simulink model "mylib_R2016b"  (R2016b)
settings: Solver=FixedStepAuto  StartTime=0.0  StopTime=10.0  RelTol=1e-3  SampleTimeConstraint=STIndependent
undefined symbols (not defined in the file or in its folder): In2, Mask_inport, Mask_outport, Out2
libraries: simulink x9
(part 1 of 2)
settings Model: Creator=Colin  LastModifiedBy=zhoutinglin
settings SimscapeCC: SimscapeNormalizeSystem=off

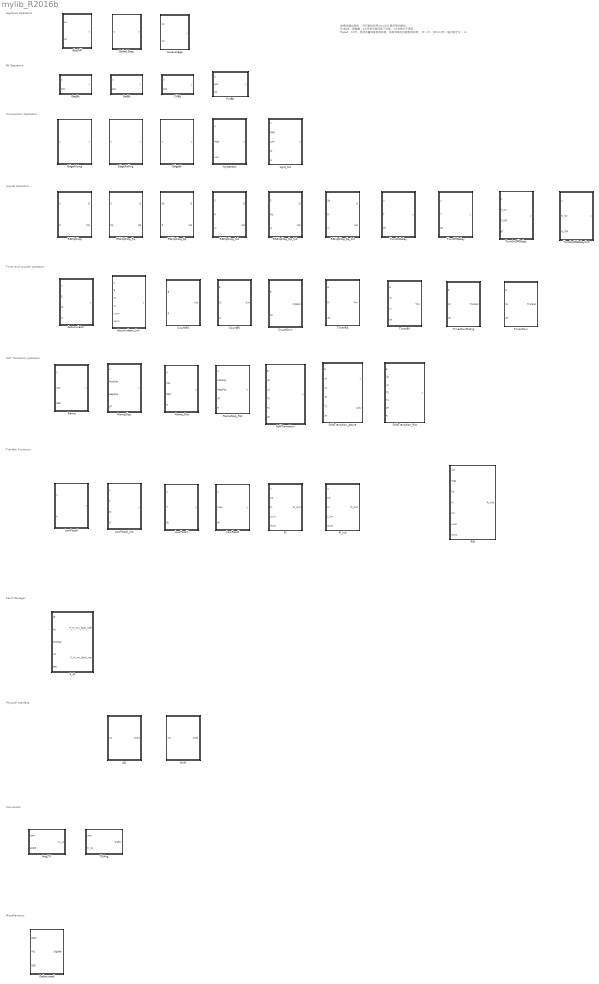
== system mylib_R2016b ==
  note: 库模块建立原则：
      | 尽可能的利用simulink里自带的模块；
      | Enable，逻辑量，=1时表示激活某个功能；=0时表示不激活，
      | Reset，=1时，将状态量恢复到初始值，或者将输出恢复到初始值；
      | IC，IV：当IC=1时，输出等于IV；
      |
      | 3.
  note: Algebraic Operators
  note: Bit Operators
  note: Comparision Operators
  note: Logical Operators
  note: Timer and counter operators
  note: Soft Transitioin operators
  note: Transfer Functions
  note: Fault Manager
  note: Physical Interface
  note: Conversion
  note: Miscellaneous
  AD : Subsystem
  AbsDiff : Subsystem
  Accumulator : Subsystem
  Accumulator_Lim : Subsystem
  Ang2Ti : Subsystem
  ClrBit : Subsystem
  CountDwn : Subsystem
  CountEV : Subsystem
  CountRE : Subsystem
  Debounced : Subsystem
  Delta1Step : Subsystem
  EdgeBi : Subsystem
  EdgeFalling : Subsystem
  EdgeRising : Subsystem
  F_M : Subsystem
  GetBit : Subsystem
  Hyst_Init : Subsystem
  Hysteresis : Subsystem
  LowPassF : Subsystem
  LowPassK : Subsystem
  LowPassK_Init : Subsystem
  LowPassT : Subsystem
  NVM : Subsystem
  PI : Subsystem
  PID : Subsystem
  PI_Init : Subsystem
  PutBit : Subsystem
  RSFilpFlop : Subsystem
  RSFilpFlop_Init : Subsystem
  RSFilpFlop_Rp : Subsystem
  RSFilpFlop_Rp_Init : Subsystem
  RSFilpFlop_Sp : Subsystem
  RSFilpFlop_Sp_Init : Subsystem
  Ramp : Subsystem
  RampSlop : Subsystem
  RampSlop_Rst : Subsystem
  Ramp_Rst : Subsystem
  SetBit : Subsystem
  SoftTransition : Subsystem
  SoftTransition_Active : Subsystem
  SoftTransition_Rst : Subsystem
  Ti2Ang : Subsystem
  TimerDwn : Subsystem
  TimerDwnRetrig : Subsystem
  TimerEV : Subsystem
  TimerRE : Subsystem
  TurnOffDelay : Subsystem
  TurnOnDelay : Subsystem
  TurnOnOffDelay : Subsystem
  TurnOnOffDelayCnt : Subsystem
  twoAverage : Subsystem

== system mylib_R2016b/AD ==
  In1 : Inport
  Out1 : Outport

== system mylib_R2016b/AbsDiff ==
  u1 : Inport
  u2 : Inport  Port=2
  Abs : Abs  RndMeth=Round  SaturateOnIntegerOverflow=on
  Subtract : Sum  Inputs=+-  RndMeth=Round  SaturateOnIntegerOverflow=on  InputSameDT=on  OutDataTypeStr=Inherit: Same as first input
  y : Outport
  wires:
  Abs/1 -> y/1
  u1/1 -> Subtract/1
  u2/1 -> Subtract/2
  Subtract/1 -> Abs/1

== system mylib_R2016b/Accumulator ==
  u : Inport
  E : Inport  Port=2  OutDataTypeStr=boolean
  IC : Inport  Port=3  OutDataTypeStr=boolean
  IV : Inport  Port=4
  Add : Sum  RndMeth=Round  SaturateOnIntegerOverflow=on  InputSameDT=on  OutDataTypeStr=Inherit: Same as first input
  Delay : Delay  DelayLength=1  InitialConditionSource=Input port  ExternalReset=Rising
      settings: InputPortMap=u0,r5,p4
  Switch : Switch  Criteria=u2 ~= 0  InputSameDT=on
  Switch1 : Switch  Criteria=u2 ~= 0  InputSameDT=on
  y : Outport
  wires:
  E/1 -> Delay/2, Switch/2
  Switch1/1 -> Delay/1, y/1
  IC/1 -> Switch1/2
  IV/1 -> Switch1/1
  Switch/1 -> Switch1/3
  u/1 -> Delay/3, Add/1
  Delay/1 -> Switch/3, Add/2
  Add/1 -> Switch/1

== system mylib_R2016b/Accumulator_Lim ==
  u : Inport
  E : Inport  Port=2  OutDataTypeStr=boolean
  IC : Inport  Port=3  OutDataTypeStr=boolean
  IV : Inport  Port=4
  LLim : Inport  Port=5
  HLim : Inport  Port=6
  Add : Sum  RndMeth=Round  SaturateOnIntegerOverflow=on  InputSameDT=on  OutDataTypeStr=Inherit: Same as first input
  Delay : Delay  DelayLength=1  InitialConditionSource=Input port  ExternalReset=Rising
      settings: InputPortMap=u0,r5,p4
  Relational Operator : RelationalOperator  Operator=<=  OutDataTypeStr=boolean  RndMeth=Simplest  InputSameDT=on
  Relational Operator1 : RelationalOperator  OutDataTypeStr=boolean  RndMeth=Simplest  InputSameDT=on
  Switch : Switch  Criteria=u2 ~= 0  InputSameDT=on
  Switch1 : Switch  Criteria=u2 ~= 0  InputSameDT=on
  Switch2 : Switch  Criteria=u2 ~= 0
  Switch3 : Switch  Criteria=u2 ~= 0
  y : Outport
  wires:
  E/1 -> Delay/2, Switch/2
  IC/1 -> Switch1/2
  IV/1 -> Switch1/1
  u/1 -> Delay/3, Add/1
  Delay/1 -> Switch/3, Add/2
  Add/1 -> Switch/1
  Relational Operator1/1 -> Switch2/2
  LLim/1 -> Switch3/1, Relational Operator/2
  Relational Operator/1 -> Switch3/2
  HLim/1 -> Relational Operator1/2, Switch2/1
  Switch2/1 -> Switch3/3
  Switch/1 -> Switch1/3
  Switch1/1 -> Switch2/3, Relational Operator1/1, Relational Operator/1
  Switch3/1 -> Delay/1, y/1

== system mylib_R2016b/Ang2Ti ==
  rpm : Inport
  angle : Inport  Port=2
  Constant : Constant  Value=1000000  OutDataTypeStr=uint32
  Constant1 : Constant  Value=6  OutDataTypeStr=uint8
  Divide : Product  Inputs=*/  OutDataTypeStr=fixdt(1,32,10)  SaturateOnIntegerOverflow=on
  Divide1 : Product  Inputs=*/  OutDataTypeStr=fixdt(1,32,10)  SaturateOnIntegerOverflow=on
  Product : Product  OutDataTypeStr=Inherit: Inherit via back propagation  SaturateOnIntegerOverflow=on
  ti_us : Outport
  wires:
  rpm/1 -> Divide/2
  Constant/1 -> Divide/1
  Divide/1 -> Divide1/1
  Constant1/1 -> Divide1/2
  Divide1/1 -> Product/1
  angle/1 -> Product/2
  Product/1 -> ti_us/1

== system mylib_R2016b/ClrBit ==
  u : Inport
  pos : Inport  Port=2  OutDataTypeStr=uint8
  Bitwise Operator : simulink/Logic and Bit Operations/Bitwise Operator  logicop=AND  UseBitMask=off  NumInputPorts=2  BitMask=bin2dec('11011001')  BitMaskRealWorld=Stored Integer
  Bitwise Operator1 : simulink/Logic and Bit Operations/Bitwise Operator  logicop=NOT  UseBitMask=off  BitMask=bin2dec('11011001')  BitMaskRealWorld=Stored Integer
  Constant2 : Constant  OutDataTypeStr=Inherit: Inherit via back propagation
  Data Type Duplicate : DataTypeDuplicate  NumInputPorts=3
  Shift Arithmetic : ArithShift  BitShiftNumberSource=Input port  BitShiftNumber=8  BitShiftDirection=Left
      settings: InputPortMap=u0,p1
  y : Outport
  wires:
  pos/1 -> Shift Arithmetic/2
  Shift Arithmetic/1 -> Bitwise Operator1/1
  Constant2/1 -> Data Type Duplicate/2, Shift Arithmetic/1
  u/1 -> Data Type Duplicate/1, Bitwise Operator/1
  Bitwise Operator/1 -> Data Type Duplicate/3, y/1
  Bitwise Operator1/1 -> Bitwise Operator/2

== system mylib_R2016b/CountDwn ==
  E : Inport  OutDataTypeStr=boolean
  SV : Inport  Port=2
  Add : Sum  Inputs=+-  RndMeth=Round  SaturateOnIntegerOverflow=on  InputSameDT=on  OutDataTypeStr=Inherit: Same as first input
  Constant : Constant  OutDataTypeStr=Inherit: Inherit via back propagation
  Constant2 : Constant  Value=0  OutDataTypeStr=Inherit: Inherit via back propagation
  Delay : Delay  DelayLength=1  InitialConditionSource=Input port  ExternalReset=Rising
      settings: InputPortMap=u0,r5,p4
  Relational Operator : RelationalOperator  Operator=<=  OutDataTypeStr=boolean  RndMeth=Simplest  InputSameDT=on
  Switch : Switch  Criteria=u2 ~= 0  InputSameDT=on
  CntEnd : Outport  OutDataTypeStr=boolean
  wires:
  Add/1 -> Switch/1
  Switch/1 -> Delay/1, Relational Operator/1
  Delay/1 -> Switch/3, Add/1
  Constant/1 -> Add/2
  SV/1 -> Delay/3
  E/1 -> Switch/2, Delay/2
  Relational Operator/1 -> CntEnd/1
  Constant2/1 -> Relational Operator/2

== system mylib_R2016b/CountEV ==
  E : Inport  OutDataTypeStr=boolean
  IC : Inport  Port=2  OutDataTypeStr=boolean
  IV : Inport  Port=3
  Add : Sum  OutDataTypeStr=Inherit: Inherit via back propagation  RndMeth=Round  SaturateOnIntegerOverflow=on  InputSameDT=on
  Constant : Constant  OutDataTypeStr=Inherit: Inherit via back propagation
  Data Type Duplicate : DataTypeDuplicate
  Switch : Switch  Criteria=u2 ~= 0  OutDataTypeStr=Inherit: Inherit via back propagation  InputSameDT=on
  Switch1 : Switch  Criteria=u2 ~= 0  OutDataTypeStr=Inherit: Inherit via back propagation  InputSameDT=on
  Unit Delay : UnitDelay  SampleTime=-1
      settings: AttributesFormatString=InitialValue=%<InitialCondition>
  Cnt : Outport
  wires:
  E/1 -> Switch/2
  Add/1 -> Switch/1
  Switch1/1 -> Data Type Duplicate/2, Unit Delay/1, Cnt/1
  IC/1 -> Switch1/2
  IV/1 -> Data Type Duplicate/1, Switch1/1
  Switch/1 -> Switch1/3
  Constant/1 -> Add/1
  Unit Delay/1 -> Switch/3, Add/2

== system mylib_R2016b/CountRE ==
  E : Inport  OutDataTypeStr=boolean
  R : Inport  Port=2  OutDataTypeStr=boolean
  Add : Sum  OutDataTypeStr=Inherit: Inherit via back propagation  SaturateOnIntegerOverflow=on  InputSameDT=on
  Constant : Constant  OutDataTypeStr=Inherit: Inherit via back propagation
  Constant2 : Constant  Value=0  OutDataTypeStr=Inherit: Inherit via back propagation
  Switch : Switch  Criteria=u2 ~= 0  OutDataTypeStr=Inherit: Inherit via back propagation  InputSameDT=on
  Switch1 : Switch  Criteria=u2 ~= 0  OutDataTypeStr=Inherit: Inherit via back propagation  InputSameDT=on
  Unit Delay : UnitDelay  SampleTime=-1
      settings: AttributesFormatString=InitialValue=%<InitialCondition>
  Cnt : Outport
  wires:
  E/1 -> Switch/2
  Add/1 -> Switch/1
  Switch1/1 -> Unit Delay/1, Cnt/1
  R/1 -> Switch1/2
  Constant2/1 -> Switch1/1
  Switch/1 -> Switch1/3
  Constant/1 -> Add/1
  Unit Delay/1 -> Switch/3, Add/2

== system mylib_R2016b/Debounced ==
  SigIn : Inport  OutDataTypeStr=boolean
  INC : Inport  Port=2
  DEC : Inport  Port=3
  Add : Sum
  Constant : Constant  Value=65535
  Constant1 : Constant  Value=0  OutDataTypeStr=boolean
  Constant2 : Constant  OutDataTypeStr=boolean
  Relational Operator : RelationalOperator  OutDataTypeStr=boolean  RndMeth=Simplest
  Subtract : Sum  Inputs=+-
  Switch : Switch  Criteria=u2 ~= 0
  Switch1 : Switch  Criteria=u2 ~= 0
  Unit Delay : UnitDelay  SampleTime=-1
      settings: AttributesFormatString=InitialValue=%<InitialCondition>
  SigDeb : Outport  OutDataTypeStr=boolean
  wires:
  SigIn/1 -> Switch/2
  Switch/1 -> Unit Delay/1, Relational Operator/1
  Constant/1 -> Relational Operator/2
  Relational Operator/1 -> Switch1/2
  Switch1/1 -> SigDeb/1
  Constant1/1 -> Switch1/3
  Constant2/1 -> Switch1/1
  INC/1 -> Add/2
  Unit Delay/1 -> Subtract/1, Add/1
  Add/1 -> Switch/1
  Subtract/1 -> Switch/3
  DEC/1 -> Subtract/2

== system mylib_R2016b/Delta1Step ==
  u : Inport
  Delay : Delay  DelayLength=1  InitialConditionSource=Input port
      settings: InputPortMap=u0,p4
  Subtract : Sum  Inputs=+-  RndMeth=Round  SaturateOnIntegerOverflow=on  InputSameDT=on  OutDataTypeStr=Inherit: Same as first input
  y : Outport
  wires:
  u/1 -> Delay/1, Delay/2, Subtract/1
  Subtract/1 -> y/1
  Delay/1 -> Subtract/2

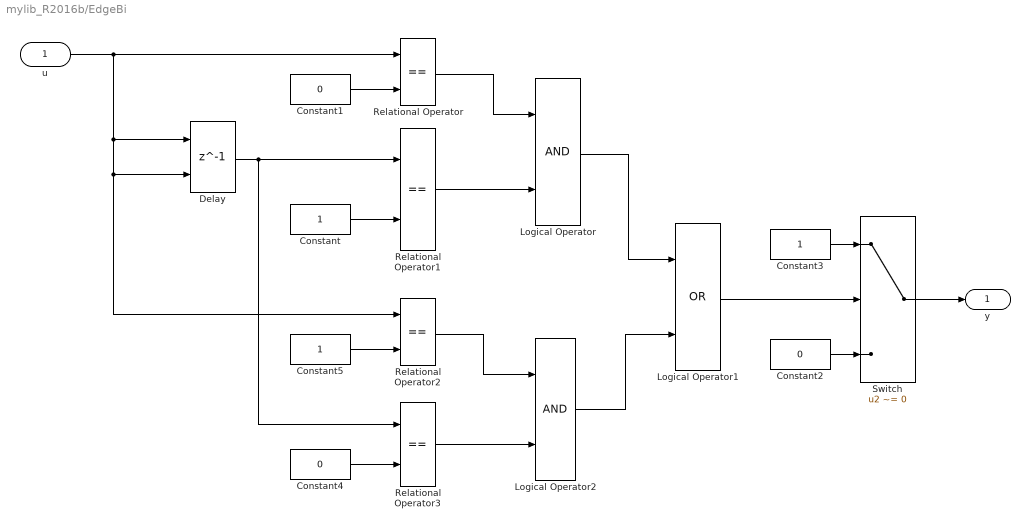
== system mylib_R2016b/EdgeBi ==
  u : Inport  OutDataTypeStr=boolean
  Constant : Constant  OutDataTypeStr=boolean
  Constant1 : Constant  Value=0  OutDataTypeStr=boolean
  Constant2 : Constant  Value=0  OutDataTypeStr=boolean
  Constant3 : Constant  OutDataTypeStr=boolean
  Constant4 : Constant  Value=0  OutDataTypeStr=boolean
  Constant5 : Constant  OutDataTypeStr=boolean
  Delay : Delay  DelayLength=1  InitialConditionSource=Input port
      settings: InputPortMap=u0,p4
  Logical Operator : Logic  AllPortsSameDT=off  OutDataTypeStr=boolean
  Logical Operator1 : Logic  Operator=OR  AllPortsSameDT=off  OutDataTypeStr=boolean
  Logical Operator2 : Logic  AllPortsSameDT=off  OutDataTypeStr=boolean
  Relational Operator{,1..3} (4 alike) : RelationalOperator  Operator===  OutDataTypeStr=boolean  RndMeth=Simplest
  Switch : Switch  Criteria=u2 ~= 0  InputSameDT=on
  y : Outport  OutDataTypeStr=boolean
  wires:
  Delay/1 -> Relational Operator3/1, Relational Operator1/1
  Switch/1 -> y/1
  Constant/1 -> Relational Operator1/2
  Constant1/1 -> Relational Operator/2
  Relational Operator1/1 -> Logical Operator/2
  Relational Operator/1 -> Logical Operator/1
  Constant2/1 -> Switch/3
  Constant3/1 -> Switch/1
  Logical Operator/1 -> Logical Operator1/1
  Logical Operator2/1 -> Logical Operator1/2
  u/1 -> Relational Operator2/1, Delay/2, Delay/1, Relational Operator/1
  Constant5/1 -> Relational Operator2/2
  Relational Operator2/1 -> Logical Operator2/1
  Constant4/1 -> Relational Operator3/2
  Relational Operator3/1 -> Logical Operator2/2
  Logical Operator1/1 -> Switch/2

== system mylib_R2016b/EdgeFalling ==
  u : Inport  OutDataTypeStr=boolean
  Constant : Constant  OutDataTypeStr=boolean
  Constant1 : Constant  Value=0  OutDataTypeStr=boolean
  Constant2 : Constant  Value=0  OutDataTypeStr=boolean
  Constant3 : Constant  OutDataTypeStr=boolean
  Delay : Delay  DelayLength=1  InitialConditionSource=Input port
      settings: InputPortMap=u0,p4
  Logical Operator : Logic  AllPortsSameDT=off  OutDataTypeStr=boolean
  Relational Operator : RelationalOperator  Operator===  OutDataTypeStr=boolean  RndMeth=Simplest
  Relational Operator1 : RelationalOperator  Operator===  OutDataTypeStr=boolean  RndMeth=Simplest
  Switch : Switch  Criteria=u2 ~= 0  InputSameDT=on
  y : Outport  OutDataTypeStr=boolean
  wires:
  Logical Operator/1 -> Switch/2
  Switch/1 -> y/1
  u/1 -> Delay/2, Delay/1, Relational Operator/1
  Constant1/1 -> Relational Operator/2
  Constant/1 -> Relational Operator1/2
  Delay/1 -> Relational Operator1/1
  Relational Operator/1 -> Logical Operator/1
  Relational Operator1/1 -> Logical Operator/2
  Constant2/1 -> Switch/3
  Constant3/1 -> Switch/1

== system mylib_R2016b/EdgeRising ==
  u : Inport  OutDataTypeStr=boolean
  Constant : Constant  Value=0  OutDataTypeStr=boolean
  Constant1 : Constant  OutDataTypeStr=boolean
  Constant2 : Constant  Value=0  OutDataTypeStr=boolean
  Constant3 : Constant  OutDataTypeStr=boolean
  Delay : Delay  DelayLength=1  InitialConditionSource=Input port
      settings: InputPortMap=u0,p4
  Logical Operator : Logic  AllPortsSameDT=off  OutDataTypeStr=boolean
  Relational Operator : RelationalOperator  Operator===  OutDataTypeStr=boolean  RndMeth=Simplest
  Relational Operator1 : RelationalOperator  Operator===  OutDataTypeStr=boolean  RndMeth=Simplest
  Switch : Switch  Criteria=u2 ~= 0  InputSameDT=on
  y : Outport  OutDataTypeStr=boolean
  wires:
  Logical Operator/1 -> Switch/2
  Switch/1 -> y/1
  u/1 -> Delay/1, Delay/2, Relational Operator/1
  Constant1/1 -> Relational Operator/2
  Constant/1 -> Relational Operator1/2
  Delay/1 -> Relational Operator1/1
  Relational Operator/1 -> Logical Operator/1
  Relational Operator1/1 -> Logical Operator/2
  Constant2/1 -> Switch/3
  Constant3/1 -> Switch/1

== system mylib_R2016b/F_M ==
  df : Inport  LibraryBlock=Mask_inport/In2  OutDataTypeStr=boolean
  frz : Inport  LibraryBlock=Mask_inport/In2  Port=2  OutDataTypeStr=boolean
  enClear : Inport  LibraryBlock=Mask_inport/In2  Port=3  OutDataTypeStr=boolean
  inc : Inport  LibraryBlock=Mask_inport/In2  Port=4  OutDataTypeStr=uint16
  dec : Inport  LibraryBlock=Mask_inport/In2  Port=5  OutDataTypeStr=uint16
  Soft : Subsystem
  rec : Subsystem
  F_M_xxx_fault_soft : Outport  LibraryBlock=Mask_outport/Out2  OutDataTypeStr=boolean  OutputWhenUnconnectedValue=0  VectorParamsAs1DForOutWhenUnconnected=off
  F_M_xxx_fault_rec : Outport  LibraryBlock=Mask_outport/Out2  Port=2  OutDataTypeStr=boolean  OutputWhenUnconnectedValue=0  VectorParamsAs1DForOutWhenUnconnected=off
  wires:
  inc/1 -> rec/4(inc)
  dec/1 -> rec/5(dec)
  Soft/1(F_M_xxx_fault_soft) -> F_M_xxx_fault_soft/1
  rec/1(F_M_xxx_fault_rec) -> F_M_xxx_fault_rec/1
  df/1 -> rec/1(df), Soft/1(df)
  frz/1 -> rec/2(frz), Soft/2(frz)
  enClear/1 -> rec/3(enClear)

== system mylib_R2016b/GetBit ==
  u : Inport
  pos : Inport  Port=2  OutDataTypeStr=uint8
  Bitwise Operator : simulink/Logic and Bit Operations/Bitwise Operator  logicop=AND  UseBitMask=off  NumInputPorts=2  BitMask=bin2dec('11011001')  BitMaskRealWorld=Stored Integer
  Compare To Zero : simulink/Logic and Bit Operations/Compare To Zero  relop=>  OutDataTypeStr=boolean  ZeroCross=off
  Constant2 : Constant  OutDataTypeStr=Inherit: Inherit via back propagation
  Data Type Duplicate : DataTypeDuplicate
  Shift Arithmetic : ArithShift  BitShiftNumberSource=Input port  BitShiftNumber=8  BitShiftDirection=Left
      settings: InputPortMap=u0,p1
  y : Outport  OutDataTypeStr=boolean
  wires:
  Compare To Zero/1 -> y/1
  u/1 -> Data Type Duplicate/1, Bitwise Operator/1
  Constant2/1 -> Data Type Duplicate/2, Shift Arithmetic/1
  Shift Arithmetic/1 -> Bitwise Operator/2
  Bitwise Operator/1 -> Compare To Zero/1
  pos/1 -> Shift Arithmetic/2

== system mylib_R2016b/Hyst_Init ==
  u : Inport
  High : Inport  Port=2
  Low : Inport  Port=3
  IC : Inport  Port=4  OutDataTypeStr=boolean
  IV : Inport  Port=5  OutDataTypeStr=boolean
  Constant : Constant  OutDataTypeStr=boolean
  Constant1 : Constant  Value=0  OutDataTypeStr=boolean
  Delay : Delay  DelayLength=1  InitialConditionSource=Input port
      settings: InputPortMap=u0,p4
  Relational Operator : RelationalOperator  Operator=>  OutDataTypeStr=boolean  RndMeth=Nearest  InputSameDT=on
  Relational Operator1 : RelationalOperator  Operator=<  OutDataTypeStr=boolean  RndMeth=Nearest  InputSameDT=on
  Switch : Switch  Criteria=u2 ~= 0  InputSameDT=on
  Switch1 : Switch  Criteria=u2 ~= 0  InputSameDT=on
  Switch2 : Switch  Criteria=u2 ~= 0  InputSameDT=on
  y : Outport  OutDataTypeStr=boolean
  wires:
  u/1 -> Relational Operator/1, Relational Operator1/1
  High/1 -> Relational Operator/2
  Relational Operator/1 -> Switch/2
  Constant/1 -> Switch/1
  Switch1/1 -> Switch/3
  Relational Operator1/1 -> Switch1/2
  Low/1 -> Relational Operator1/2
  Constant1/1 -> Switch1/1
  Switch/1 -> Switch2/3
  Delay/1 -> Switch1/3
  IV/1 -> Switch2/1, Delay/2
  IC/1 -> Switch2/2
  Switch2/1 -> Delay/1, y/1

== system mylib_R2016b/Hysteresis ==
  u : Inport
  High : Inport  Port=2
  Low : Inport  Port=3
  Constant : Constant  OutDataTypeStr=boolean
  Constant1 : Constant  Value=0  OutDataTypeStr=boolean
  Delay : Delay  DelayLength=1  InitialCondition=0
      settings: AttributesFormatString=InitialValue=%<InitialCondition>
  Relational Operator : RelationalOperator  Operator=>  OutDataTypeStr=boolean  RndMeth=Nearest  InputSameDT=on
  Relational Operator1 : RelationalOperator  Operator=<  OutDataTypeStr=boolean  RndMeth=Nearest  InputSameDT=on
  Switch : Switch  Criteria=u2 ~= 0  InputSameDT=on
  Switch1 : Switch  Criteria=u2 ~= 0  InputSameDT=on
  y : Outport  OutDataTypeStr=boolean
  wires:
  u/1 -> Relational Operator/1, Relational Operator1/1
  High/1 -> Relational Operator/2
  Relational Operator/1 -> Switch/2
  Constant/1 -> Switch/1
  Switch1/1 -> Switch/3
  Relational Operator1/1 -> Switch1/2
  Low/1 -> Relational Operator1/2
  Constant1/1 -> Switch1/1
  Switch/1 -> y/1, Delay/1
  Delay/1 -> Switch1/3

== system mylib_R2016b/LowPassF ==
  u : Inport
  Freq : Inport  Port=2
  dt : Inport  Port=3
  Constant : Constant  Value=6.2831852  OutDataTypeStr=fixdt(1,16,2^-12,0)
  Delay : Delay  DelayLength=1  InitialConditionSource=Input port
      settings: InputPortMap=u0,p4
  Product : Product  RndMeth=Round  SaturateOnIntegerOverflow=on  OutDataTypeStr=Inherit: Same as first input
  Product1 : Product  OutDataTypeStr=fixdt(1,16,2^-12,0)  RndMeth=Round  SaturateOnIntegerOverflow=on
  Product2 : Product  OutDataTypeStr=fixdt(1,16,2^-12,0)  RndMeth=Round  SaturateOnIntegerOverflow=on
  Subtract1 : Sum  Inputs=+-  RndMeth=Round  SaturateOnIntegerOverflow=on  InputSameDT=on  OutDataTypeStr=Inherit: Same as first input
  Sum : Sum  Inputs=+|+  SaturateOnIntegerOverflow=on  InputSameDT=on  OutDataTypeStr=Inherit: Same as first input
  fi([0	0.003	0.0039	0.0051	0.0066	0.0086	0.0113	0.0147	0.0191	0.0248	0.0322	0.0419	0.0542	0.0702	0.0905	0.1164	0.149	0.1898	0.2401	0.301	0.3732	0.4563	0.5483	0.6453	0.7413	0.8285	0.8997	0.9502	1],1,16,2^-14,0) : Lookup_n-D  NumberOfTableDimensions=1  BreakpointsForDimension1=|  BreakpointsForDimension1DataTypeStr=Inherit: Inherit from 'Breakpoint data'  Table="fi([0\t0.003\t0.0039\t0.0051\t0.0066\t0.0086\t0.0113\t0.0147\t0.0191\t0.0248\t0.0322\t0.0419\t0.0542\t0.0702\t0.0905\t0.1164\t0.149\t0.1898\t0.2401\t0.301\t0.3732\t0.4563\t0.5483\t0.6453\t0.7413\t0.8285\t0.8997\t0.9502\t1],1,16,2^-14,0)"  TableDataTypeStr=Inherit: Inherit from 'Table data'  ExtrapMethod=Clip  InternalRulePriority=Speed  OutDataTypeStr=Inherit: Inherit from 'Table data'  RndMeth=Round  SaturateOnIntegerOverflow=on  InputSameDT=on
      | fi([0	0.003	0.0039	0.0051	0.0067	0.0087	0.0113	0.0148	0.0193	0.0251	0.0328	0.0428	0.0558	0.0727	0.0949	0.1237	0.1614	0.2105	0.2746	0.3581	0.4671	0.6093	0.7947	1.0365	1.352	1.7634	2.3	3	7.5
      | ],1,16,2^-12,0)
  y : Outport
  wires:
  Delay/1 -> Subtract1/2, Sum/2
  Product/1 -> Sum/1
  Sum/1 -> Delay/1, y/1
  Subtract1/1 -> Product/1
  u/1 -> Delay/2, Subtract1/1
  Freq/1 -> Product1/1
  Product2/1 -> fi([0	0.003	0.0039	0.0051	0.0066	0.0086	0.0113	0.0147	0.0191	0.0248	0.0322	0.0419	0.0542	0.0702	0.0905	0.1164	0.149	0.1898	0.2401	0.301	0.3732	0.4563	0.5483	0.6453	0.7413	0.8285	0.8997	0.9502	1],1,16,2^-14,0)/1
  fi([0	0.003	0.0039	0.0051	0.0066	0.0086	0.0113	0.0147	0.0191	0.0248	0.0322	0.0419	0.0542	0.0702	0.0905	0.1164	0.149	0.1898	0.2401	0.301	0.3732	0.4563	0.5483	0.6453	0.7413	0.8285	0.8997	0.9502	1],1,16,2^-14,0)/1 -> Product/2
  dt/1 -> Product1/2
  Constant/1 -> Product2/1
  Product1/1 -> Product2/2

== system mylib_R2016b/LowPassK ==
  u : Inport
  K : Inport  Port=2
  Delay : Delay  DelayLength=1  InitialConditionSource=Input port
      settings: InputPortMap=u0,p4
  Product : Product  RndMeth=Round  SaturateOnIntegerOverflow=on  OutDataTypeStr=Inherit: Same as first input
  Subtract1 : Sum  Inputs=+-  RndMeth=Round  SaturateOnIntegerOverflow=on  InputSameDT=on  OutDataTypeStr=Inherit: Same as first input
  Sum : Sum  Inputs=+|+  SaturateOnIntegerOverflow=on  InputSameDT=on  OutDataTypeStr=Inherit: Same as first input
  y : Outport
  wires:
  u/1 -> Delay/2, Subtract1/1
  Delay/1 -> Sum/2, Subtract1/2
  Product/1 -> Sum/1
  Sum/1 -> Delay/1, y/1
  Subtract1/1 -> Product/1
  K/1 -> Product/2

== system mylib_R2016b/LowPassK_Init ==
  u : Inport
  K : Inport  Port=2
  IC : Inport  Port=3
  IV : Inport  Port=4
  Delay : Delay  DelayLength=1  InitialConditionSource=Input port
      settings: InputPortMap=u0,p4
  Product : Product  RndMeth=Round  SaturateOnIntegerOverflow=on  OutDataTypeStr=Inherit: Same as first input
  Subtract1 : Sum  Inputs=+-  RndMeth=Round  SaturateOnIntegerOverflow=on  InputSameDT=on  OutDataTypeStr=Inherit: Same as first input
  Sum : Sum  Inputs=+|+  SaturateOnIntegerOverflow=on  InputSameDT=on  OutDataTypeStr=Inherit: Same as first input
  Switch : Switch  Criteria=u2 ~= 0  RndMeth=Round  InputSameDT=on
  y : Outport
  wires:
  Switch/1 -> Delay/1, y/1
  IC/1 -> Switch/2
  IV/1 -> Switch/1
  Subtract1/1 -> Product/1
  Delay/1 -> Sum/2, Subtract1/2
  u/1 -> Delay/2, Subtract1/1
  Sum/1 -> Switch/3
  Product/1 -> Sum/1
  K/1 -> Product/2

== system mylib_R2016b/LowPassT ==
  u : Inport
  T : Inport  Port=2
  dt : Inport  Port=3
  Delay : Delay  DelayLength=1  InitialConditionSource=Input port
      settings: InputPortMap=u0,p4
  Divide : Product  Inputs=*/  OutDataTypeStr=fixdt(1,16,2^-12,0)  SaturateOnIntegerOverflow=on
  Product : Product  RndMeth=Round  SaturateOnIntegerOverflow=on  OutDataTypeStr=Inherit: Same as first input
  Subtract1 : Sum  Inputs=+-  RndMeth=Round  SaturateOnIntegerOverflow=on  InputSameDT=on  OutDataTypeStr=Inherit: Same as first input
  Sum : Sum  Inputs=+|+  SaturateOnIntegerOverflow=on  InputSameDT=on  OutDataTypeStr=Inherit: Same as first input
  fi([0	0.003	0.0039	0.0051	0.0066	0.0086	0.0113	0.0147	0.0191	0.0248	0.0322	0.0419	0.0542	0.0702	0.0905	0.1164	0.149	0.1898	0.2401	0.301	0.3732	0.4563	0.5483	0.6453	0.7413	0.8285	0.8997	0.9502	1],1,16,2^-14,0) : Lookup_n-D  NumberOfTableDimensions=1  BreakpointsForDimension1=|  BreakpointsForDimension1DataTypeStr=Inherit: Inherit from 'Breakpoint data'  Table="fi([0\t0.003\t0.0039\t0.0051\t0.0066\t0.0086\t0.0113\t0.0147\t0.0191\t0.0248\t0.0322\t0.0419\t0.0542\t0.0702\t0.0905\t0.1164\t0.149\t0.1898\t0.2401\t0.301\t0.3732\t0.4563\t0.5483\t0.6453\t0.7413\t0.8285\t0.8997\t0.9502\t1],1,16,2^-14,0)"  TableDataTypeStr=Inherit: Inherit from 'Table data'  ExtrapMethod=Clip  InternalRulePriority=Speed  OutDataTypeStr=Inherit: Inherit from 'Table data'  RndMeth=Round  SaturateOnIntegerOverflow=on  InputSameDT=on
      | fi([0	0.003	0.0039	0.0051	0.0067	0.0087	0.0113	0.0148	0.0193	0.0251	0.0328	0.0428	0.0558	0.0727	0.0949	0.1237	0.1614	0.2105	0.2746	0.3581	0.4671	0.6093	0.7947	1.0365	1.352	1.7634	2.3	3	7.5
      | ],1,16,2^-12,0)
  y : Outport
  wires:
  Delay/1 -> Subtract1/2, Sum/2
  Product/1 -> Sum/1
  Sum/1 -> Delay/1, y/1
  Subtract1/1 -> Product/1
  u/1 -> Delay/2, Subtract1/1
  dt/1 -> Divide/1
  T/1 -> Divide/2
  Divide/1 -> fi([0	0.003	0.0039	0.0051	0.0066	0.0086	0.0113	0.0147	0.0191	0.0248	0.0322	0.0419	0.0542	0.0702	0.0905	0.1164	0.149	0.1898	0.2401	0.301	0.3732	0.4563	0.5483	0.6453	0.7413	0.8285	0.8997	0.9502	1],1,16,2^-14,0)/1
  fi([0	0.003	0.0039	0.0051	0.0066	0.0086	0.0113	0.0147	0.0191	0.0248	0.0322	0.0419	0.0542	0.0702	0.0905	0.1164	0.149	0.1898	0.2401	0.301	0.3732	0.4563	0.5483	0.6453	0.7413	0.8285	0.8997	0.9502	1],1,16,2^-14,0)/1 -> Product/2

== system mylib_R2016b/NVM ==
  In1 : Inport
  Out1 : Outport

== system mylib_R2016b/PI ==
  u : Inport
  Kp : Inport  Port=2
  Ki : Inport  Port=3
  LLim : Inport  Port=4
  HLim : Inport  Port=5
  Add : Sum  SaturateOnIntegerOverflow=on
  Add1 : Sum
  Product : Product
  Product1 : Product
  Relational Operator : RelationalOperator  Operator=<=  OutDataTypeStr=boolean  RndMeth=Simplest  InputSameDT=on
  Relational Operator1 : RelationalOperator  OutDataTypeStr=boolean  RndMeth=Simplest  InputSameDT=on
  Switch : Switch  Criteria=u2 ~= 0
  Switch1 : Switch  Criteria=u2 ~= 0
  Unit Delay : UnitDelay  SampleTime=-1
      settings: AttributesFormatString=InitialValue=%<InitialCondition>
  PI_Out : Outport
  wires:
  u/1 -> Product/1, Product1/1
  Kp/1 -> Product/2
  Ki/1 -> Product1/2
  Product1/1 -> Add/1
  Add/1 -> Add1/2, Unit Delay/1
  Unit Delay/1 -> Add/2
  Product/1 -> Add1/1
  Add1/1 -> Relational Operator/1, Switch/3, Relational Operator1/1
  HLim/1 -> Relational Operator1/2, Switch/1
  LLim/1 -> Switch1/1, Relational Operator/2
  Relational Operator/1 -> Switch1/2
  Relational Operator1/1 -> Switch/2
  Switch/1 -> Switch1/3
  Switch1/1 -> PI_Out/1

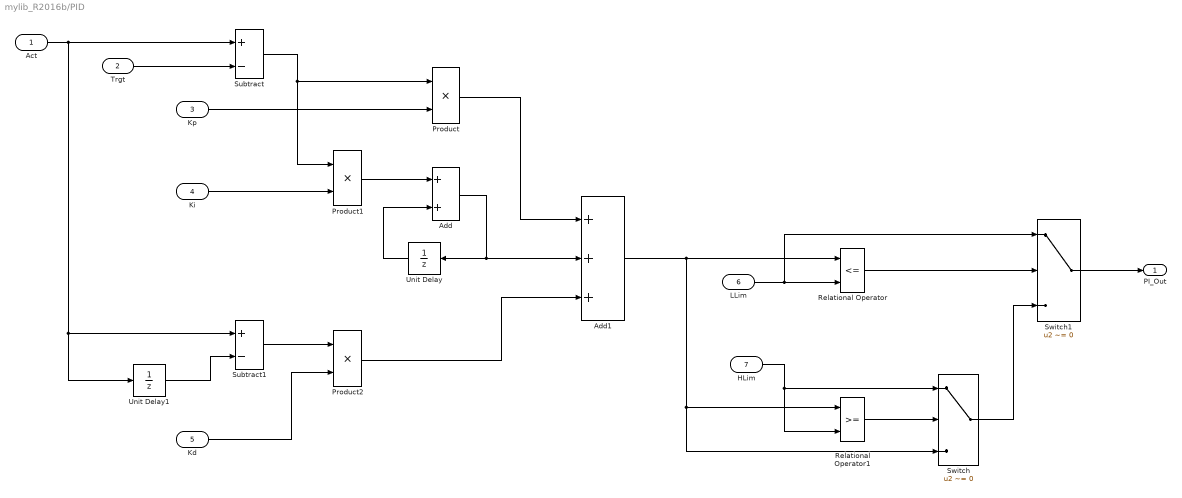
== system mylib_R2016b/PID ==
  Act : Inport
  Trgt : Inport  Port=2
  Kp : Inport  Port=3
  Ki : Inport  Port=4
  Kd : Inport  Port=5
  LLim : Inport  Port=6
  HLim : Inport  Port=7
  Add : Sum
  Add1 : Sum  Inputs=+++
  Product : Product
  Product1 : Product
  Product2 : Product
  Relational Operator : RelationalOperator  Operator=<=  OutDataTypeStr=boolean  RndMeth=Simplest  InputSameDT=on
  Relational Operator1 : RelationalOperator  OutDataTypeStr=boolean  RndMeth=Simplest  InputSameDT=on
  Subtract : Sum  Inputs=+-
  Subtract1 : Sum  Inputs=+-
  Switch : Switch  Criteria=u2 ~= 0
  Switch1 : Switch  Criteria=u2 ~= 0
  Unit Delay : UnitDelay  SampleTime=-1
      settings: AttributesFormatString=InitialValue=%<InitialCondition>
  Unit Delay1 : UnitDelay  SampleTime=-1
      settings: AttributesFormatString=InitialValue=%<InitialCondition>
  PI_Out : Outport
  wires:
  Kp/1 -> Product/2
  Ki/1 -> Product1/2
  Product1/1 -> Add/1
  Add/1 -> Unit Delay/1, Add1/2
  Unit Delay/1 -> Add/2
  Product/1 -> Add1/1
  Add1/1 -> Switch/3, Relational Operator1/1, Relational Operator/1
  HLim/1 -> Relational Operator1/2, Switch/1
  LLim/1 -> Switch1/1, Relational Operator/2
  Relational Operator/1 -> Switch1/2
  Relational Operator1/1 -> Switch/2
  Switch/1 -> Switch1/3
  Switch1/1 -> PI_Out/1
  Act/1 -> Unit Delay1/1, Subtract1/1, Subtract/1
  Trgt/1 -> Subtract/2
  Subtract/1 -> Product1/1, Product/1
  Unit Delay1/1 -> Subtract1/2
  Subtract1/1 -> Product2/1
  Kd/1 -> Product2/2
  Product2/1 -> Add1/3

== system mylib_R2016b/PI_Init ==
  u : Inport
  Kp : Inport  Port=2
  Ki : Inport  Port=3
  LLim : Inport  Port=4
  HLim : Inport  Port=5
  Add : Sum
  Add1 : Sum
  Product : Product
  Product1 : Product
  Relational Operator : RelationalOperator  Operator=<=  OutDataTypeStr=boolean  RndMeth=Simplest  InputSameDT=on
  Relational Operator1 : RelationalOperator  OutDataTypeStr=boolean  RndMeth=Simplest  InputSameDT=on
  Switch : Switch  Criteria=u2 ~= 0
  Switch1 : Switch  Criteria=u2 ~= 0
  Unit Delay : UnitDelay  SampleTime=-1
      settings: AttributesFormatString=InitialValue=%<InitialCondition>
  PI_Out : Outport
  wires:
  u/1 -> Product/1, Product1/1
  Kp/1 -> Product/2
  Ki/1 -> Product1/2
  Product1/1 -> Add/1
  Add/1 -> Add1/2, Unit Delay/1
  Unit Delay/1 -> Add/2
  Product/1 -> Add1/1
  Add1/1 -> Relational Operator/1, Switch/3, Relational Operator1/1
  HLim/1 -> Relational Operator1/2, Switch/1
  LLim/1 -> Switch1/1, Relational Operator/2
  Relational Operator/1 -> Switch1/2
  Relational Operator1/1 -> Switch/2
  Switch/1 -> Switch1/3
  Switch1/1 -> PI_Out/1

== system mylib_R2016b/PutBit ==
  u : Inport
  pos : Inport  Port=2  OutDataTypeStr=uint8
  bit : Inport  Port=3  OutDataTypeStr=boolean
  Bitwise Operator : simulink/Logic and Bit Operations/Bitwise Operator  logicop=OR  UseBitMask=off  NumInputPorts=2  BitMask=bin2dec('11011001')  BitMaskRealWorld=Stored Integer
  Bitwise Operator1 : simulink/Logic and Bit Operations/Bitwise Operator  logicop=AND  UseBitMask=off  NumInputPorts=2  BitMask=bin2dec('11011001')  BitMaskRealWorld=Stored Integer
  Bitwise Operator2 : simulink/Logic and Bit Operations/Bitwise Operator  logicop=NOT  UseBitMask=off  BitMask=bin2dec('11011001')  BitMaskRealWorld=Stored Integer
  Constant2 : Constant  OutDataTypeStr=Inherit: Inherit via back propagation
  Data Type Duplicate : DataTypeDuplicate  NumInputPorts=3
  Shift Arithmetic : ArithShift  BitShiftNumberSource=Input port  BitShiftNumber=8  BitShiftDirection=Left
      settings: InputPortMap=u0,p1
  Switch : Switch  Criteria=u2 ~= 0  RndMeth=Round  InputSameDT=on
  y : Outport
  wires:
  pos/1 -> Shift Arithmetic/2
  Constant2/1 -> Data Type Duplicate/2, Shift Arithmetic/1
  Shift Arithmetic/1 -> Bitwise Operator2/1, Bitwise Operator/2
  bit/1 -> Switch/2
  Bitwise Operator/1 -> Switch/1
  u/1 -> Data Type Duplicate/1, Bitwise Operator1/1, Bitwise Operator/1
  Bitwise Operator2/1 -> Bitwise Operator1/2
  Bitwise Operator1/1 -> Switch/3
  Switch/1 -> Data Type Duplicate/3, y/1

== system mylib_R2016b/RSFilpFlop ==
  note: S
      | R
      | Q
      | NQ
      |
      | 0
      | 1
      | 0
      | 1
      |
      | 1
      | 0
      | 1
      | 0
      |
      | 0
      | 0
      | Qn-1
      | !Qn-1
      |
      | 1
      | 1
      | 0
      | 0
  S : Inport  OutDataTypeStr=boolean
  R : Inport  Port=2  OutDataTypeStr=boolean
  Constant : Constant  Value=0  OutDataTypeStr=boolean
  Constant1 : Constant  OutDataTypeStr=boolean
  Constant2 : Constant  Value=0  OutDataTypeStr=boolean
  Constant3 : Constant  OutDataTypeStr=boolean
  Logical Operator : Logic  Operator=NOT  AllPortsSameDT=off  OutDataTypeStr=boolean
  Switch{,1..3} (4 alike) : Switch  Criteria=u2 ~= 0
  Unit Delay : UnitDelay  SampleTime=-1
      settings: AttributesFormatString=InitialValue=%<InitialCondition>
  Q : Outport  OutDataTypeStr=boolean
  NQ : Outport  Port=2  OutDataTypeStr=boolean
  wires:
  R/1 -> Switch3/2, Switch/2
  Constant/1 -> Switch/1
  Switch/1 -> Unit Delay/1, Q/1
  S/1 -> Switch2/2, Switch1/2
  Constant1/1 -> Switch1/1
  Switch1/1 -> Switch/3
  Unit Delay/1 -> Switch1/3, Logical Operator/1
  Switch2/1 -> NQ/1
  Constant2/1 -> Switch2/1
  Switch3/1 -> Switch2/3
  Constant3/1 -> Switch3/1
  Logical Operator/1 -> Switch3/3

== system mylib_R2016b/RSFilpFlop_Init ==
  note: S
      | R
      | Q
      | NQ
      |
      | 0
      | 1
      | 0
      | 1
      |
      | 1
      | 0
      | 1
      | 0
      |
      | 0
      | 0
      | Qn-1
      | !Qn-1
      |
      | 1
      | 1
      | 0
      | 0
  S : Inport  OutDataTypeStr=boolean
  R : Inport  Port=2  OutDataTypeStr=boolean
  IV : Inport  Port=3
  Constant : Constant  Value=0  OutDataTypeStr=boolean
  Constant1 : Constant  OutDataTypeStr=boolean
  Constant2 : Constant  Value=0  OutDataTypeStr=boolean
  Constant3 : Constant  OutDataTypeStr=boolean
  Delay : Delay  DelayLength=1  InitialConditionSource=Input port
      settings: InputPortMap=u0,p4
  Logical Operator : Logic  Operator=NOT  AllPortsSameDT=off  OutDataTypeStr=boolean
  Switch{,1..3} (4 alike) : Switch  Criteria=u2 ~= 0
  Q : Outport  OutDataTypeStr=boolean
  NQ : Outport  Port=2  OutDataTypeStr=boolean
  wires:
  R/1 -> Switch3/2, Switch/2
  Constant/1 -> Switch/1
  Switch/1 -> Delay/1, Q/1
  S/1 -> Switch2/2, Switch1/2
  Constant1/1 -> Switch1/1
  Switch1/1 -> Switch/3
  Delay/1 -> Switch1/3, Logical Operator/1
  Switch2/1 -> NQ/1
  Constant2/1 -> Switch2/1
  Switch3/1 -> Switch2/3
  Constant3/1 -> Switch3/1
  Logical Operator/1 -> Switch3/3
  IV/1 -> Delay/2

== system mylib_R2016b/RSFilpFlop_Rp ==
  note: S
      | R
      | Q
      | NQ
      |
      | 0
      | 1
      | 0
      | 1
      |
      | 1
      | 0
      | 1
      | 0
      |
      | 0
      | 0
      | Qn-1
      | !Qn-1
      |
      | 1
      | 1
      | 0
      | 1
  S : Inport  OutDataTypeStr=boolean
  Rp : Inport  Port=2  OutDataTypeStr=boolean
  Constant : Constant  Value=0  OutDataTypeStr=boolean
  Constant1 : Constant  OutDataTypeStr=boolean
  Logical Operator : Logic  Operator=NOT  AllPortsSameDT=off  OutDataTypeStr=boolean
  Switch : Switch  Criteria=u2 ~= 0
  Switch1 : Switch  Criteria=u2 ~= 0
  Unit Delay : UnitDelay  SampleTime=-1
      settings: AttributesFormatString=InitialValue=%<InitialCondition>
  Q : Outport  OutDataTypeStr=boolean
  NQ : Outport  Port=2  OutDataTypeStr=boolean
  wires:
  Rp/1 -> Switch/2
  Constant/1 -> Switch/1
  Switch/1 -> Logical Operator/1, Unit Delay/1, Q/1
  S/1 -> Switch1/2
  Constant1/1 -> Switch1/1
  Switch1/1 -> Switch/3
  Unit Delay/1 -> Switch1/3
  Logical Operator/1 -> NQ/1

== system mylib_R2016b/RSFilpFlop_Rp_Init ==
  note: S
      | R
      | Q
      | NQ
      |
      | 0
      | 1
      | 0
      | 1
      |
      | 1
      | 0
      | 1
      | 0
      |
      | 0
      | 0
      | Qn-1
      | !Qn-1
      |
      | 1
      | 1
      | 0
      | 1
  S : Inport  OutDataTypeStr=boolean
  Rp : Inport  Port=2  OutDataTypeStr=boolean
  IV : Inport  Port=3
  Constant : Constant  Value=0  OutDataTypeStr=boolean
  Constant1 : Constant  OutDataTypeStr=boolean
  Delay : Delay  DelayLength=1  InitialConditionSource=Input port
      settings: InputPortMap=u0,p4
  Logical Operator : Logic  Operator=NOT  AllPortsSameDT=off  OutDataTypeStr=boolean
  Switch : Switch  Criteria=u2 ~= 0
  Switch1 : Switch  Criteria=u2 ~= 0
  Q : Outport  OutDataTypeStr=boolean
  NQ : Outport  Port=2  OutDataTypeStr=boolean
  wires:
  Rp/1 -> Switch/2
  Constant/1 -> Switch/1
  Switch/1 -> Delay/1, Logical Operator/1, Q/1
  S/1 -> Switch1/2
  Constant1/1 -> Switch1/1
  Switch1/1 -> Switch/3
  Delay/1 -> Switch1/3
  Logical Operator/1 -> NQ/1
  IV/1 -> Delay/2

== system mylib_R2016b/RSFilpFlop_Sp ==
  note: S
      | R
      | Q
      | NQ
      |
      | 0
      | 1
      | 0
      | 1
      |
      | 1
      | 0
      | 1
      | 0
      |
      | 0
      | 0
      | Qn-1
      | !Qn-1
      |
      | 1
      | 1
      | 1
      | 0
  Sp : Inport  OutDataTypeStr=boolean
  R : Inport  Port=2  OutDataTypeStr=boolean
  Constant : Constant  OutDataTypeStr=boolean
  Constant1 : Constant  Value=0  OutDataTypeStr=boolean
  Logical Operator : Logic  Operator=NOT  AllPortsSameDT=off  OutDataTypeStr=boolean
  Switch : Switch  Criteria=u2 ~= 0
  Switch1 : Switch  Criteria=u2 ~= 0
  Unit Delay : UnitDelay  SampleTime=-1
      settings: AttributesFormatString=InitialValue=%<InitialCondition>
  Q : Outport  OutDataTypeStr=boolean
  NQ : Outport  Port=2  OutDataTypeStr=boolean
  wires:
  Constant/1 -> Switch/1
  Switch/1 -> Logical Operator/1, Unit Delay/1, Q/1
  Constant1/1 -> Switch1/1
  Switch1/1 -> Switch/3
  Unit Delay/1 -> Switch1/3
  Logical Operator/1 -> NQ/1
  Sp/1 -> Switch/2
  R/1 -> Switch1/2

== system mylib_R2016b/RSFilpFlop_Sp_Init ==
  note: S
      | R
      | Q
      | NQ
      |
      | 0
      | 1
      | 0
      | 1
      |
      | 1
      | 0
      | 1
      | 0
      |
      | 0
      | 0
      | Qn-1
      | !Qn-1
      |
      | 1
      | 1
      | 1
      | 0
  Sp : Inport  OutDataTypeStr=boolean
  R : Inport  Port=2  OutDataTypeStr=boolean
  IV : Inport  Port=3
  Constant : Constant  OutDataTypeStr=boolean
  Constant1 : Constant  Value=0  OutDataTypeStr=boolean
  Delay : Delay  DelayLength=1  InitialConditionSource=Input port
      settings: InputPortMap=u0,p4
  Logical Operator : Logic  Operator=NOT  AllPortsSameDT=off  OutDataTypeStr=boolean
  Switch : Switch  Criteria=u2 ~= 0
  Switch1 : Switch  Criteria=u2 ~= 0
  Q : Outport  OutDataTypeStr=boolean
  NQ : Outport  Port=2  OutDataTypeStr=boolean
  wires:
  Constant/1 -> Switch/1
  Switch/1 -> Delay/1, Logical Operator/1, Q/1
  Constant1/1 -> Switch1/1
  Switch1/1 -> Switch/3
  Delay/1 -> Switch1/3
  Logical Operator/1 -> NQ/1
  Sp/1 -> Switch/2
  R/1 -> Switch1/2
  IV/1 -> Delay/2

== system mylib_R2016b/Ramp ==
  note: y=y_1+Step, Step被限制在[-DEC INC]内
  u : Inport
  INC : Inport  Port=2
  DEC : Inport  Port=3
  Add1 : Sum  RndMeth=Round  SaturateOnIntegerOverflow=on  InputSameDT=on  OutDataTypeStr=Inherit: Same as first input
  Delay1 : Delay  DelayLength=1  InitialConditionSource=Input port
      settings: InputPortMap=u0,p4
  Max : MinMax  Inputs=2  InputSameDT=on
  Max1 : MinMax  Function=max  Inputs=2  InputSameDT=on
  Subtract : Sum  Inputs=+-  RndMeth=Round  SaturateOnIntegerOverflow=on  InputSameDT=on  OutDataTypeStr=Inherit: Same as first input
  Unary Minus : UnaryMinus
  y : Outport
  wires:
  DEC/1 -> Unary Minus/1
  Add1/1 -> y/1, Delay1/1
  Delay1/1 -> Add1/1, Subtract/2
  u/1 -> Delay1/2, Subtract/1
  Subtract/1 -> Max/1
  INC/1 -> Max/2
  Max/1 -> Max1/1
  Unary Minus/1 -> Max1/2
  Max1/1 -> Add1/2

== system mylib_R2016b/RampSlop ==
  note: y=y_1+Step, Step被限制在[-NegSlop*dT PosSlop*dT]内
  u : Inport
  PosSlop : Inport  Port=2
  NegSlop : Inport  Port=3
  dT : Inport  Port=4
  Add1 : Sum  RndMeth=Round  SaturateOnIntegerOverflow=on  InputSameDT=on  OutDataTypeStr=Inherit: Same as first input
  Delay1 : Delay  DelayLength=1  InitialConditionSource=Input port
      settings: InputPortMap=u0,p4
  Max : MinMax  Inputs=2  InputSameDT=on
  Max1 : MinMax  Function=max  Inputs=2  InputSameDT=on
  Product : Product  OutDataTypeStr=Inherit: Inherit via back propagation  RndMeth=Round  SaturateOnIntegerOverflow=on
  Product1 : Product  OutDataTypeStr=Inherit: Inherit via back propagation  RndMeth=Round  SaturateOnIntegerOverflow=on
  Subtract : Sum  Inputs=+-  RndMeth=Round  SaturateOnIntegerOverflow=on  InputSameDT=on  OutDataTypeStr=Inherit: Same as first input
  Unary Minus : UnaryMinus
  y : Outport
  wires:
  Add1/1 -> y/1, Delay1/1
  u/1 -> Delay1/2, Subtract/1
  Unary Minus/1 -> Max1/2
  Product/1 -> Max/2
  Subtract/1 -> Max/1
  Delay1/1 -> Add1/1, Subtract/2
  Product1/1 -> Unary Minus/1
  Max/1 -> Max1/1
  Max1/1 -> Add1/2
  PosSlop/1 -> Product/1
  dT/1 -> Product1/2, Product/2
  NegSlop/1 -> Product1/1

== system mylib_R2016b/RampSlop_Rst ==
  note: y=y_1+Step, Step被限制在[-NegSlop*dT PosSlop*dT]内
  u : Inport
  PosSlop : Inport  Port=2
  NegSlop : Inport  Port=3
  dT : Inport  Port=4
  R : Inport  Port=5  OutDataTypeStr=boolean
  Add1 : Sum  RndMeth=Round  SaturateOnIntegerOverflow=on  InputSameDT=on  OutDataTypeStr=Inherit: Same as first input
  Delay1 : Delay  DelayLength=1  InitialConditionSource=Input port
      settings: InputPortMap=u0,p4
  Max : MinMax  Inputs=2  InputSameDT=on
  Max1 : MinMax  Function=max  Inputs=2  InputSameDT=on
  Product : Product  OutDataTypeStr=Inherit: Inherit via back propagation  RndMeth=Round  SaturateOnIntegerOverflow=on
  Product1 : Product  OutDataTypeStr=Inherit: Inherit via back propagation  RndMeth=Round  SaturateOnIntegerOverflow=on
  Subtract : Sum  Inputs=+-  RndMeth=Round  SaturateOnIntegerOverflow=on  InputSameDT=on  OutDataTypeStr=Inherit: Same as first input
  Switch : Switch  Criteria=u2 ~= 0  InputSameDT=on
  Unary Minus : UnaryMinus
  y : Outport
  wires:
  u/1 -> Switch/1, Delay1/2, Subtract/1
  Unary Minus/1 -> Max1/2
  Product/1 -> Max/2
  Subtract/1 -> Max/1
  Delay1/1 -> Add1/1, Subtract/2
  Product1/1 -> Unary Minus/1
  Max/1 -> Max1/1
  Max1/1 -> Add1/2
  PosSlop/1 -> Product/1
  dT/1 -> Product1/2, Product/2
  NegSlop/1 -> Product1/1
  Add1/1 -> Switch/3
  R/1 -> Switch/2
  Switch/1 -> Delay1/1, y/1

== system mylib_R2016b/Ramp_Rst ==
  note: y=y_1+Step, Step被限制在[-DEC INC]内
  u : Inport
  INC : Inport  Port=2
  DEC : Inport  Port=3
  R : Inport  Port=4  OutDataTypeStr=boolean
  Add1 : Sum  RndMeth=Round  SaturateOnIntegerOverflow=on  InputSameDT=on  OutDataTypeStr=Inherit: Same as first input
  Delay1 : Delay  DelayLength=1  InitialConditionSource=Input port
      settings: InputPortMap=u0,p4
  Max : MinMax  Inputs=2  InputSameDT=on
  Max1 : MinMax  Function=max  Inputs=2  InputSameDT=on
  Subtract : Sum  Inputs=+-  RndMeth=Round  SaturateOnIntegerOverflow=on  InputSameDT=on  OutDataTypeStr=Inherit: Same as first input
  Switch : Switch  Criteria=u2 ~= 0  InputSameDT=on
  Unary Minus : UnaryMinus
  y : Outport
  wires:
  DEC/1 -> Unary Minus/1
  Delay1/1 -> Add1/1, Subtract/2
  u/1 -> Delay1/2, Switch/1, Subtract/1
  Subtract/1 -> Max/1
  INC/1 -> Max/2
  Max/1 -> Max1/1
  Unary Minus/1 -> Max1/2
  Max1/1 -> Add1/2
  Switch/1 -> Delay1/1, y/1
  R/1 -> Switch/2
  Add1/1 -> Switch/3

== system mylib_R2016b/SetBit ==
  u : Inport
  pos : Inport  Port=2  OutDataTypeStr=uint8
  Bitwise Operator : simulink/Logic and Bit Operations/Bitwise Operator  logicop=OR  UseBitMask=off  NumInputPorts=2  BitMask=bin2dec('11011001')  BitMaskRealWorld=Stored Integer
  Constant2 : Constant  OutDataTypeStr=Inherit: Inherit via back propagation
  Data Type Duplicate : DataTypeDuplicate  NumInputPorts=3
  Shift Arithmetic : ArithShift  BitShiftNumberSource=Input port  BitShiftNumber=8  BitShiftDirection=Left
      settings: InputPortMap=u0,p1
  y : Outport
  wires:
  Shift Arithmetic/1 -> Bitwise Operator/2
  Constant2/1 -> Data Type Duplicate/2, Shift Arithmetic/1
  u/1 -> Data Type Duplicate/1, Bitwise Operator/1
  Bitwise Operator/1 -> Data Type Duplicate/3, y/1
  pos/1 -> Shift Arithmetic/2

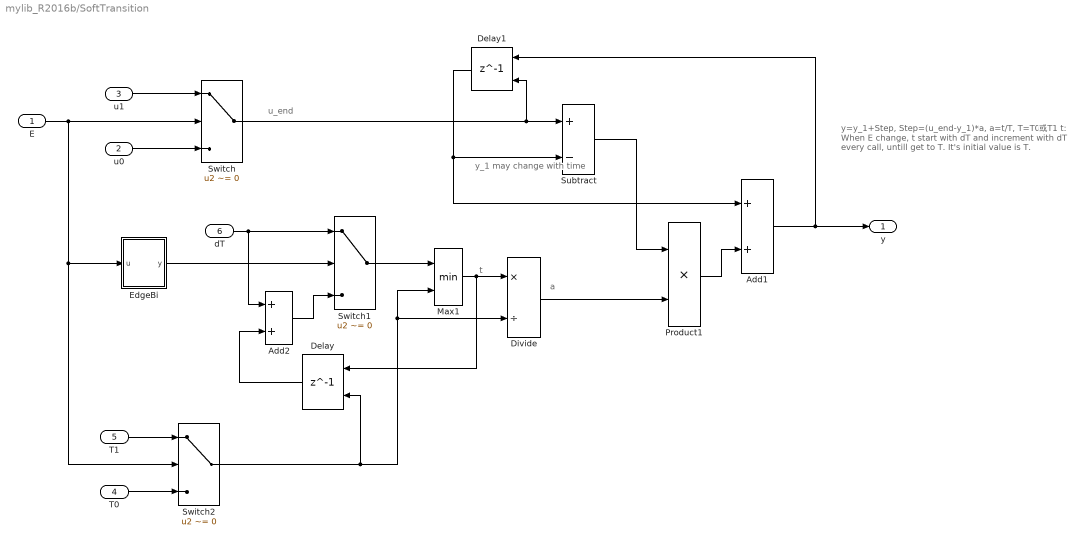
== system mylib_R2016b/SoftTransition ==
  note: y_1 may change
      |  with time
  note: t
  note: a
  note: u_end
  note: y=y_1+Step, Step=(u_end-y_1)*a, a=t/T, T=T0或T1
      | t: When E change, t start with dT and increment with dT every call, untill get to T. It's initial value is T.
  E : Inport
  u0 : Inport  Port=2
  u1 : Inport  Port=3
  T0 : Inport  Port=4
  T1 : Inport  Port=5
  dT : Inport  Port=6
  Add1 : Sum  RndMeth=Round  SaturateOnIntegerOverflow=on  InputSameDT=on  OutDataTypeStr=Inherit: Same as first input
  Add2 : Sum  RndMeth=Round  SaturateOnIntegerOverflow=on  InputSameDT=on  OutDataTypeStr=Inherit: Same as first input
  Delay : Delay  DelayLength=1  InitialConditionSource=Input port
      settings: InputPortMap=u0,p4
  Delay1 : Delay  DelayLength=1  InitialConditionSource=Input port
      settings: InputPortMap=u0,p4
  Divide : Product  Inputs=*/  OutDataTypeStr=fixdt(1,16,2^-14,0)  RndMeth=Round  SaturateOnIntegerOverflow=on  InputSameDT=on
  EdgeBi : Subsystem
  Max1 : MinMax  Inputs=2  InputSameDT=on
  Product1 : Product  RndMeth=Round  SaturateOnIntegerOverflow=on  OutDataTypeStr=Inherit: Same as first input
  Subtract : Sum  Inputs=+-  RndMeth=Round  SaturateOnIntegerOverflow=on  InputSameDT=on  OutDataTypeStr=Inherit: Same as first input
  Switch : Switch  Criteria=u2 ~= 0  InputSameDT=on
  Switch1 : Switch  Criteria=u2 ~= 0  InputSameDT=on
  Switch2 : Switch  Criteria=u2 ~= 0  InputSameDT=on
  y : Outport
  wires:
  E/1 -> Switch2/2, EdgeBi/1(u), Switch/2
  u1/1 -> Switch/1
  u0/1 -> Switch/3
  Switch2/1 -> Divide/2, Max1/2, Delay/2
  Delay/1 -> Add2/2
  T1/1 -> Switch2/1
  T0/1 -> Switch2/3
  Max1/1 -> Delay/1, Divide/1
  Divide/1 -> Product1/2
  Add1/1 -> y/1, Delay1/1
  Product1/1 -> Add1/2
  Delay1/1 -> Subtract/2, Add1/1
  Switch/1 -> Delay1/2, Subtract/1
  Subtract/1 -> Product1/1
  Add2/1 -> Switch1/3
  EdgeBi/1(y) -> Switch1/2
  dT/1 -> Add2/1, Switch1/1
  Switch1/1 -> Max1/1

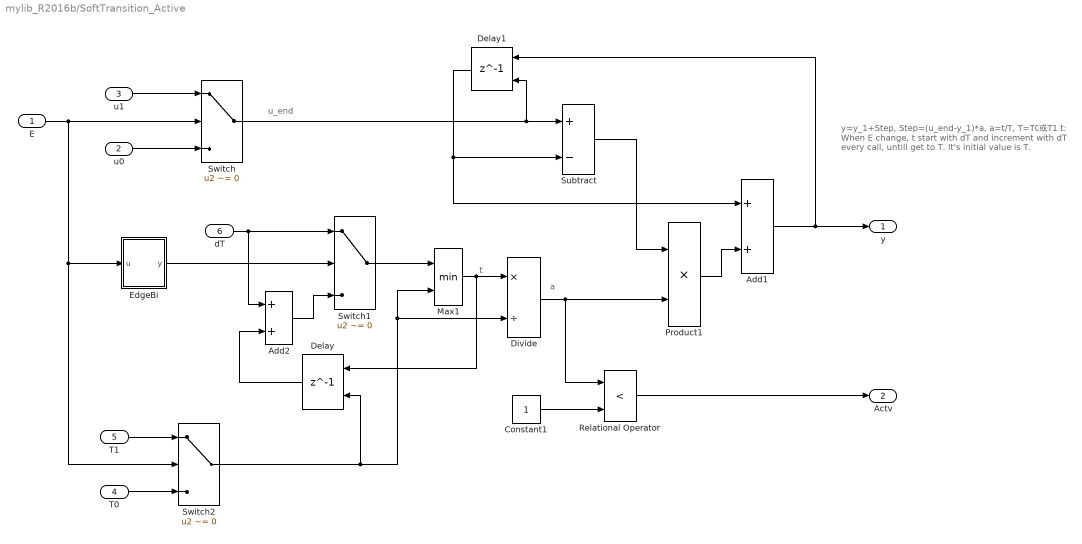
== system mylib_R2016b/SoftTransition_Active ==
  note: t
  note: a
  note: u_end
  note: y=y_1+Step, Step=(u_end-y_1)*a, a=t/T, T=T0或T1
      | t: When E change, t start with dT and increment with dT every call, untill get to T. It's initial value is T.
  E : Inport
  u0 : Inport  Port=2
  u1 : Inport  Port=3
  T0 : Inport  Port=4
  T1 : Inport  Port=5
  dT : Inport  Port=6
  Add1 : Sum  RndMeth=Round  SaturateOnIntegerOverflow=on  InputSameDT=on  OutDataTypeStr=Inherit: Same as first input
  Add2 : Sum  RndMeth=Round  SaturateOnIntegerOverflow=on  InputSameDT=on  OutDataTypeStr=Inherit: Same as first input
  Constant1 : Constant  OutDataTypeStr=Inherit: Inherit via back propagation
  Delay : Delay  DelayLength=1  InitialConditionSource=Input port
      settings: InputPortMap=u0,p4
  Delay1 : Delay  DelayLength=1  InitialConditionSource=Input port
      settings: InputPortMap=u0,p4
  Divide : Product  Inputs=*/  OutDataTypeStr=fixdt(1,16,2^-14,0)  RndMeth=Round  SaturateOnIntegerOverflow=on  InputSameDT=on
  EdgeBi : Subsystem
  Max1 : MinMax  Inputs=2  InputSameDT=on
  Product1 : Product  RndMeth=Round  SaturateOnIntegerOverflow=on  OutDataTypeStr=Inherit: Same as first input
  Relational Operator : RelationalOperator  Operator=<  OutDataTypeStr=boolean  RndMeth=Simplest  InputSameDT=on
  Subtract : Sum  Inputs=+-  RndMeth=Round  SaturateOnIntegerOverflow=on  InputSameDT=on  OutDataTypeStr=Inherit: Same as first input
  Switch : Switch  Criteria=u2 ~= 0  InputSameDT=on
  Switch1 : Switch  Criteria=u2 ~= 0  InputSameDT=on
  Switch2 : Switch  Criteria=u2 ~= 0  InputSameDT=on
  y : Outport
  Actv : Outport  Port=2
  wires:
  E/1 -> Switch2/2, EdgeBi/1(u), Switch/2
  u1/1 -> Switch/1
  u0/1 -> Switch/3
  Switch2/1 -> Divide/2, Max1/2, Delay/2
  Delay/1 -> Add2/2
  T1/1 -> Switch2/1
  T0/1 -> Switch2/3
  Max1/1 -> Delay/1, Divide/1
  Divide/1 -> Relational Operator/1, Product1/2
  Add1/1 -> y/1, Delay1/1
  Product1/1 -> Add1/2
  Delay1/1 -> Subtract/2, Add1/1
  Switch/1 -> Delay1/2, Subtract/1
  Subtract/1 -> Product1/1
  Add2/1 -> Switch1/3
  EdgeBi/1(y) -> Switch1/2
  dT/1 -> Add2/1, Switch1/1
  Switch1/1 -> Max1/1
  Constant1/1 -> Relational Operator/2
  Relational Operator/1 -> Actv/1

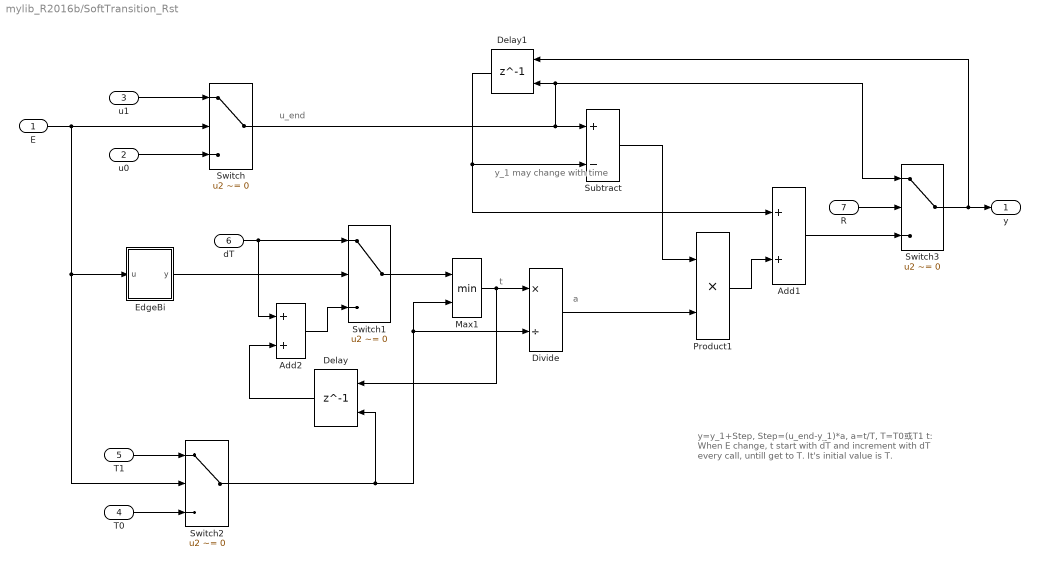
== system mylib_R2016b/SoftTransition_Rst ==
  note: y_1 may change
      |  with time
  note: t
  note: a
  note: u_end
  note: y=y_1+Step, Step=(u_end-y_1)*a, a=t/T, T=T0或T1
      | t: When E change, t start with dT and increment with dT every call, untill get to T. It's initial value is T.
  E : Inport
  u0 : Inport  Port=2
  u1 : Inport  Port=3
  T0 : Inport  Port=4
  T1 : Inport  Port=5
  dT : Inport  Port=6
  R : Inport  Port=7  OutDataTypeStr=boolean
  Add1 : Sum  RndMeth=Round  SaturateOnIntegerOverflow=on  InputSameDT=on  OutDataTypeStr=Inherit: Same as first input
  Add2 : Sum  RndMeth=Round  SaturateOnIntegerOverflow=on  InputSameDT=on  OutDataTypeStr=Inherit: Same as first input
  Delay : Delay  DelayLength=1  InitialConditionSource=Input port
      settings: InputPortMap=u0,p4
  Delay1 : Delay  DelayLength=1  InitialConditionSource=Input port
      settings: InputPortMap=u0,p4
  Divide : Product  Inputs=*/  OutDataTypeStr=fixdt(1,16,2^-14,0)  RndMeth=Round  SaturateOnIntegerOverflow=on  InputSameDT=on
  EdgeBi : Subsystem
  Max1 : MinMax  Inputs=2  InputSameDT=on
  Product1 : Product  RndMeth=Round  SaturateOnIntegerOverflow=on  OutDataTypeStr=Inherit: Same as first input
  Subtract : Sum  Inputs=+-  RndMeth=Round  SaturateOnIntegerOverflow=on  InputSameDT=on  OutDataTypeStr=Inherit: Same as first input
  Switch{,1..3} (4 alike) : Switch  Criteria=u2 ~= 0  InputSameDT=on
  y : Outport
  wires:
  E/1 -> Switch2/2, EdgeBi/1(u), Switch/2
  u1/1 -> Switch/1
  u0/1 -> Switch/3
  Switch2/1 -> Divide/2, Max1/2, Delay/2
  Delay/1 -> Add2/2
  T1/1 -> Switch2/1
  T0/1 -> Switch2/3
  Max1/1 -> Delay/1, Divide/1
  Divide/1 -> Product1/2
  Product1/1 -> Add1/2
  Delay1/1 -> Subtract/2, Add1/1
  Switch/1 -> Subtract/1, Switch3/1, Delay1/2
  Subtract/1 -> Product1/1
  Add2/1 -> Switch1/3
  EdgeBi/1(y) -> Switch1/2
  dT/1 -> Add2/1, Switch1/1
  Switch1/1 -> Max1/1
  R/1 -> Switch3/2
  Add1/1 -> Switch3/3
  Switch3/1 -> Delay1/1, y/1

== system mylib_R2016b/Ti2Ang ==
  rpm : Inport
  ti_us : Inport  Port=2
  Constant : Constant  Value=1000000  OutDataTypeStr=uint32
  Constant1 : Constant  Value=6  OutDataTypeStr=uint8
  Divide : Product  Inputs=*/  OutDataTypeStr=fixdt(1,32,10)  SaturateOnIntegerOverflow=on
  Product : Product  OutDataTypeStr=Inherit: Inherit via back propagation  SaturateOnIntegerOverflow=on
  Product1 : Product  OutDataTypeStr=fixdt(1,32,10)  SaturateOnIntegerOverflow=on
  angle : Outport
  wires:
  Product/1 -> angle/1
  Constant1/1 -> Product/2
  ti_us/1 -> Product1/1
  rpm/1 -> Product1/2
  Product1/1 -> Divide/1
  Constant/1 -> Divide/2
  Divide/1 -> Product/1

== system mylib_R2016b/TimerDwn ==
  E : Inport  OutDataTypeStr=boolean
  SV : Inport  Port=2
  dT : Inport  Port=3
  Add : Sum  Inputs=+-  RndMeth=Round  SaturateOnIntegerOverflow=on  InputSameDT=on  OutDataTypeStr=Inherit: Same as first input
  Constant1 : Constant  Value=0  OutDataTypeStr=Inherit: Inherit via back propagation
  Constant2 : Constant  Value=0  OutDataTypeStr=Inherit: Inherit via back propagation
  Delay : Delay  DelayLength=1  InitialConditionSource=Input port
      settings: InputPortMap=u0,p4
  EdgeRising : Subsystem
  Logical Operator : Logic  AllPortsSameDT=off  OutDataTypeStr=boolean
  Relational Operator : RelationalOperator  Operator=<=  OutDataTypeStr=boolean  RndMeth=Simplest  InputSameDT=on
  Relational Operator1 : RelationalOperator  Operator=<=  OutDataTypeStr=boolean  RndMeth=Simplest  InputSameDT=on
  Switch : Switch  Criteria=u2 ~= 0  InputSameDT=on
  Switch1 : Switch  Criteria=u2 ~= 0  InputSameDT=on
  TmrEnd : Outport  OutDataTypeStr=boolean
  wires:
  Add/1 -> Relational Operator1/1, Switch/1
  Delay/1 -> Switch/3, Add/1
  Relational Operator/1 -> TmrEnd/1
  SV/1 -> Delay/2, Switch1/1
  dT/1 -> Add/2
  Constant2/1 -> Relational Operator/2
  Constant1/1 -> Relational Operator1/2
  Relational Operator1/1 -> Logical Operator/2
  E/1 -> EdgeRising/1(u), Switch/2
  Logical Operator/1 -> Switch1/2
  Switch/1 -> Switch1/3
  Switch1/1 -> Relational Operator/1, Delay/1
  EdgeRising/1(y) -> Logical Operator/1
